simulink library "INT_APP_Plaus12"  (R2016b)
settings: Solver=VariableStepAuto  StartTime=0.0  StopTime=10.0  RelTol=1e-3
settings Model: Creator=Administrator  LastModifiedBy=Administrator

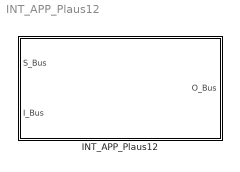
== system INT_APP_Plaus12 ==
  INT_APP_Plaus12 : Subsystem

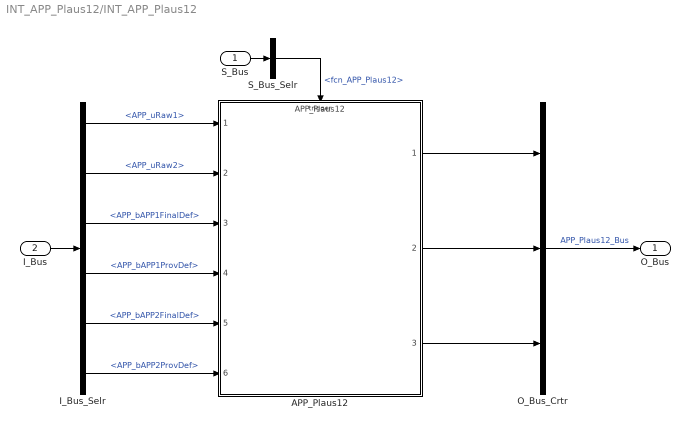
== system INT_APP_Plaus12/INT_APP_Plaus12 ==
  S_Bus : Inport
  I_Bus : Inport  Port=2
  APP_Plaus12 : ModelReference  ModelNameDialog=APP_Plaus12  SimulationMode=Normal  ModelReferenceVersion=1.23  TriggerPortName=function  TriggerPortTriggerType=function-call  TriggerPortStatesWhenEnabling=held
  I_Bus_Selr : BusSelector  OutputSignals=APP_uRaw1,APP_uRaw2,APP_bAPP1FinalDef,APP_bAPP1ProvDef,APP_bAPP2FinalDef,APP_bAPP2ProvDef
  O_Bus_Crtr : BusCreator  Inputs=3
  S_Bus_Selr : BusSelector  OutputSignals=fcn_APP_Plaus12
  O_Bus : Outport
  wires:
  S_Bus_Selr/1 -> APP_Plaus12/Trigger  "<fcn_APP_Plaus12>"
  S_Bus/1 -> S_Bus_Selr/1
  I_Bus/1 -> I_Bus_Selr/1
  I_Bus_Selr/1 -> APP_Plaus12/1  "<APP_uRaw1>"
  I_Bus_Selr/2 -> APP_Plaus12/2  "<APP_uRaw2>"
  I_Bus_Selr/3 -> APP_Plaus12/3  "<APP_bAPP1FinalDef>"
  I_Bus_Selr/4 -> APP_Plaus12/4  "<APP_bAPP1ProvDef>"
  I_Bus_Selr/5 -> APP_Plaus12/5  "<APP_bAPP2FinalDef>"
  I_Bus_Selr/6 -> APP_Plaus12/6  "<APP_bAPP2ProvDef>"
  O_Bus_Crtr/1 -> O_Bus/1  "APP_Plaus12_Bus"
  APP_Plaus12/1 -> O_Bus_Crtr/1
  APP_Plaus12/2 -> O_Bus_Crtr/2
  APP_Plaus12/3 -> O_Bus_Crtr/3
